simulink model "ex5"  (R2016b)
settings: Solver=ode23s  StartTime=0.0  StopTime=0.2  RelTol=1e-3
InitFcn:
  | ex5LIN_param
values from neighbouring files (symbols this model uses):
  A = [0 1; 0 -(dm/Jeq + Km*Kemf/(R*Jeq))]    [Lab3.m]    (also in Lab3_1.m; Lab3_2.m; Lab3_2_discrete_disg.m; Lab3_3.m)
  A1 = A3    (= 0.00180641577581)    [ex5LIN_param.m]    (also in param.m)
  A2 = A3    (= 0.00180641577581)    [ex5LIN_param.m]    (also in param.m)
  B = [0; Km/(R*Jeq)]    [Lab3.m]    (also in Lab3_1.m; Lab3_2.m; Lab3_2_discrete_disg.m; Lab3_3.m)
  beta = 2e9    (= 2000000000)    [ex5LIN_param.m]    (also in param.m)
  C = [1/n 0; 0 1/n]    [Lab3.m]    (also in Lab3_1.m; Lab3_2.m; Lab3_2_discrete_disg.m; Lab3_3.m)
  Cf1 = Cf    (= 6.32245521535e-13)    [ex5LIN_param.m]    (also in param.m)
  Cf2 = Cf    (= 6.32245521535e-13)    [ex5LIN_param.m]    (also in param.m)
  d = 0.001    [ex5LIN_param.m]    (also in param.m)
  D0 = zeros(3,2)    [ex5LIN.m]
  D_FBv = D_temp{1,1}    [ex5PID.m]
  D_FFv = D_temp{1,1}    [ex5PID.m]
  df = 200    [ex5LIN_param.m]    (also in param.m)
  fe0 = feINI(z)    [ex5LIN.m]
  m = 100    [ex5LIN_param.m]    (also in param.m)
  N_FBv = N_temp{1,1}    [ex5PID.m]
  N_FFv = N_temp{1,1}    [ex5PID.m]
  p1q0 = p1qINI(z)    [ex5LIN.m]
  p2q0 = p2qINI(z)    [ex5LIN.m]
  Ps = 20e6    (= 20000000)    [ex5LIN_param.m]    (also in param.m)
  Pt = 0    [ex5LIN_param.m]    (also in param.m)
  Rv = 1e-4    (= 0.0001)    [ex5LIN_param.m]    (also in param.m)
  smax = 0.7    [ex5LIN_param.m]    (also in param.m)
  vn = -0.01    [ex5LIN_param.m]    (also in param.m)
  vp = 0.01    [ex5LIN_param.m]    (also in param.m)
  vq0 = vqINI(z)    [ex5LIN.m]
  xvq0 = xvqINI(z)    [ex5LIN.m]
undefined symbols (not defined in the file or in its folder): D_C, D_FF, I_C, I_FF, K_C, K_FF, P_C, P_FF
libraries: simulink x4
settings Model: Creator=Philipp  LastModifiedBy=Philipp

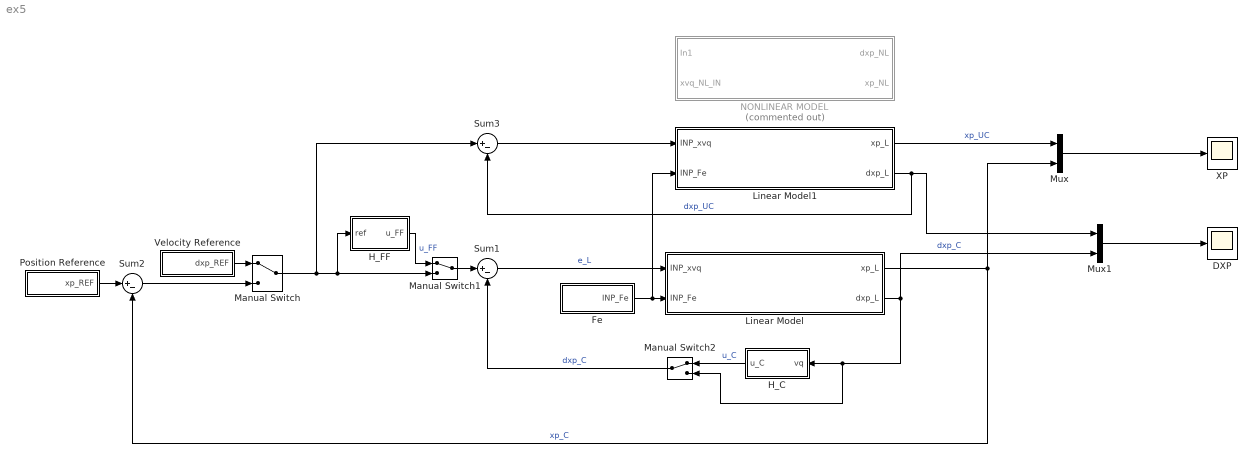
== system ex5 ==
  DXP : Scope
  Fe : Subsystem
  H_C : Subsystem
  H_FF : Subsystem
  Linear Model : Subsystem
  Linear Model1 : Subsystem
  Manual Switch : ManualSwitch
  Manual Switch1 : ManualSwitch
  Manual Switch2 : ManualSwitch
  Mux : Mux  Inputs=2
  Mux1 : Mux  Inputs=2
  NONLINEAR MODEL : Subsystem  Commented=on
  Position Reference : Subsystem
  Sum1 : Sum  Inputs=|+-
  Sum2 : Sum  Inputs=|+-
  Sum3 : Sum  Inputs=|+-
  Velocity Reference : Subsystem
  XP : Scope
  wires:
  H_FF/1(u_FF) -> Manual Switch1/1  "u_FF"
  H_C/1(u_C) -> Manual Switch2/1  "u_C"
  Sum2/1 -> Manual Switch/2
  Manual Switch/1 -> Sum3/1, H_FF/1(ref), Manual Switch1/2
  Manual Switch2/1 -> Sum1/2  "dxp_C"
  Manual Switch1/1 -> Sum1/1
  Position Reference/1(xp_REF) -> Sum2/1
  Velocity Reference/1(dxp_REF) -> Manual Switch/1
  Fe/1(INP_Fe) -> Linear Model1/2(INP_Fe), Linear Model/2(INP_Fe)
  Linear Model/2(dxp_L) -> Manual Switch2/2, H_C/1(vq), Mux1/2  "dxp_C"
  Linear Model/1(xp_L) -> Mux/2, Sum2/2  "xp_C"
  Sum1/1 -> Linear Model/1(INP_xvq)  "e_L"
  Linear Model1/1(xp_L) -> Mux/1  "xp_UC"
  Linear Model1/2(dxp_L) -> Sum3/2, Mux1/1  "dxp_UC"
  Mux1/1 -> DXP/1
  Mux/1 -> XP/1
  Sum3/1 -> Linear Model1/1(INP_xvq)

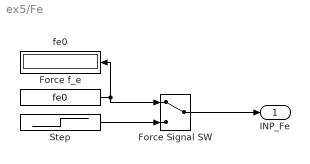
== system ex5/Fe ==
  Force Signal SW : ManualSwitch
  Force f_e : Constant  Value=fe0
  Step : Step  Time=0.12  After=0  SampleTime=0
  fe0 : Display
  INP_Fe : Outport
  wires:
  Force Signal SW/1 -> INP_Fe/1
  Force f_e/1 -> fe0/1, Force Signal SW/1
  Step/1 -> Force Signal SW/2

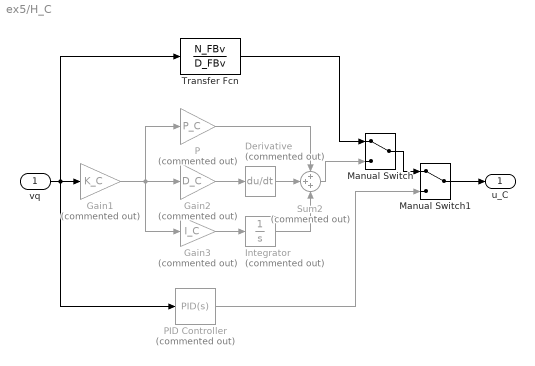
== system ex5/H_C ==
  vq : Inport
  Derivative : Derivative  Commented=on  CoefficientInTFapproximation=T_LPC
  Gain1 : Gain  Commented=on  Gain=K_C
  Gain2 : Gain  Commented=on  Gain=D_C
  Gain3 : Gain  Commented=on  Gain=I_C
  Integrator : Integrator  Commented=on
  Manual Switch : ManualSwitch
  Manual Switch1 : ManualSwitch
  P : Gain  Commented=on  Gain=P_C
  PID Controller : simulink/Continuous/PID Controller  Commented=on  Controller=PID  TimeDomain=Continuous-time  SampleTime=-1  IntegratorMethod=Forward Euler  FilterMethod=Forward Euler  Form=Parallel  UseFilter=on  ControllerParametersSource=internal  P=1  I=1  D=0  N=100  InitialConditionSource=internal  InitialConditionForIntegrator=0  InitialConditionForFilter=0  ExternalReset=none  LimitOutput=off  UpperSaturationLimit=inf  LowerSaturationLimit=-inf  LinearizeAsGain=on  AntiWindupMode=none  Kb=1  TrackingMode=off  Kt=1  PParamMin=[]  PParamMax=[]  IParamMin=[]  IParamMax=[]  DParamMin=[]  DParamMax=[]  NParamMin=[]  NParamMax=[]  KbParamMin=[]  KbParamMax=[]  KtParamMin=[]  KtParamMax=[]  POutMin=[]  POutMax=[]  IOutMin=[]  IOutMax=[]  DOutMin=[]  DOutMax=[]  NOutMin=[]  NOutMax=[]  KbOutMin=[]  KbOutMax=[]  KtOutMin=[]  KtOutMax=[]  IntegratorOutMin=[]  IntegratorOutMax=[]  FilterOutMin=[]  FilterOutMax=[]  SumOutMin=[]  SumOutMax=[]  SumI1OutMin=[]  SumI1OutMax=[]  SumI2OutMin=[]  SumI2OutMax=[]  SumI3OutMin=[]  SumI3OutMax=[]  SumDOutMin=[]  SumDOutMax=[]  SaturationOutMin=[]  SaturationOutMax=[]  IntegratorContinuousStateAttributes=''  IntegratorStateMustResolveToSignalObject=off  IntegratorRTWStateStorageClass=Auto  FilterContinuousStateAttributes=''  FilterStateMustResolveToSignalObject=off  FilterRTWStateStorageClass=Auto  DifferentiatorICPrevScaledInput=0  DifferentiatorOutMin=[]  DifferentiatorOutMax=[]
  Sum2 : Sum  Commented=on  Inputs=+++
  Transfer Fcn : TransferFcn  Numerator=N_FBv  Denominator=D_FBv
  u_C : Outport
  wires:
  Gain3/1 -> Integrator/1
  vq/1 -> PID Controller/1, Transfer Fcn/1, Gain1/1
  P/1 -> Sum2/1
  Derivative/1 -> Sum2/2
  Gain2/1 -> Derivative/1
  Integrator/1 -> Sum2/3
  Gain1/1 -> Gain3/1, Gain2/1, P/1
  Manual Switch1/1 -> u_C/1
  Manual Switch/1 -> Manual Switch1/1
  Transfer Fcn/1 -> Manual Switch/1
  Sum2/1 -> Manual Switch/2
  PID Controller/1 -> Manual Switch1/2

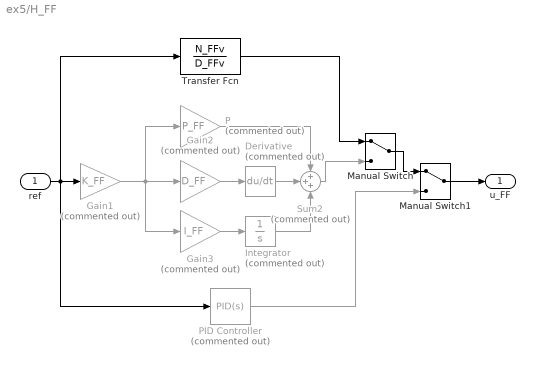
== system ex5/H_FF ==
  ref : Inport
  Derivative : Derivative  Commented=on  CoefficientInTFapproximation=T_LPFF
  Gain1 : Gain  Commented=on  Gain=K_FF
  Gain2 : Gain  Commented=on  Gain=D_FF
  Gain3 : Gain  Commented=on  Gain=I_FF
  Integrator : Integrator  Commented=on
  Manual Switch : ManualSwitch
  Manual Switch1 : ManualSwitch
  P : Gain  Commented=on  Gain=P_FF
  PID Controller : simulink/Continuous/PID Controller  Commented=on  Controller=PID  TimeDomain=Continuous-time  SampleTime=-1  IntegratorMethod=Forward Euler  FilterMethod=Forward Euler  Form=Parallel  UseFilter=on  ControllerParametersSource=internal  P=1  I=1  D=0  N=100  InitialConditionSource=internal  InitialConditionForIntegrator=0  InitialConditionForFilter=0  ExternalReset=none  LimitOutput=off  UpperSaturationLimit=inf  LowerSaturationLimit=-inf  LinearizeAsGain=on  AntiWindupMode=none  Kb=1  TrackingMode=off  Kt=1  PParamMin=[]  PParamMax=[]  IParamMin=[]  IParamMax=[]  DParamMin=[]  DParamMax=[]  NParamMin=[]  NParamMax=[]  KbParamMin=[]  KbParamMax=[]  KtParamMin=[]  KtParamMax=[]  POutMin=[]  POutMax=[]  IOutMin=[]  IOutMax=[]  DOutMin=[]  DOutMax=[]  NOutMin=[]  NOutMax=[]  KbOutMin=[]  KbOutMax=[]  KtOutMin=[]  KtOutMax=[]  IntegratorOutMin=[]  IntegratorOutMax=[]  FilterOutMin=[]  FilterOutMax=[]  SumOutMin=[]  SumOutMax=[]  SumI1OutMin=[]  SumI1OutMax=[]  SumI2OutMin=[]  SumI2OutMax=[]  SumI3OutMin=[]  SumI3OutMax=[]  SumDOutMin=[]  SumDOutMax=[]  SaturationOutMin=[]  SaturationOutMax=[]  IntegratorContinuousStateAttributes=''  IntegratorStateMustResolveToSignalObject=off  IntegratorRTWStateStorageClass=Auto  FilterContinuousStateAttributes=''  FilterStateMustResolveToSignalObject=off  FilterRTWStateStorageClass=Auto  DifferentiatorICPrevScaledInput=0  DifferentiatorOutMin=[]  DifferentiatorOutMax=[]
  Sum2 : Sum  Commented=on  Inputs=+++
  Transfer Fcn : TransferFcn  Numerator=N_FFv  Denominator=D_FFv
  u_FF : Outport
  wires:
  Gain3/1 -> Integrator/1
  ref/1 -> PID Controller/1, Transfer Fcn/1, Gain1/1
  P/1 -> Sum2/1
  Derivative/1 -> Sum2/2
  Gain2/1 -> Derivative/1
  Integrator/1 -> Sum2/3
  Gain1/1 -> Gain3/1, Gain2/1, P/1
  Manual Switch1/1 -> u_FF/1
  Manual Switch/1 -> Manual Switch1/1
  Transfer Fcn/1 -> Manual Switch/1
  Sum2/1 -> Manual Switch/2
  PID Controller/1 -> Manual Switch1/2

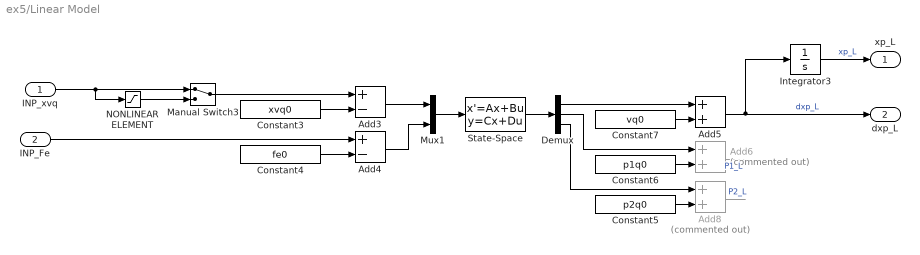
== system ex5/Linear Model ==
  INP_xvq : Inport
  INP_Fe : Inport  Port=2
  Add3 : Sum  Inputs=+-
  Add4 : Sum  Inputs=+-
  Add5 : Sum
  Add6 : Sum  Commented=on
  Add8 : Sum  Commented=on
  Constant3 : Constant  Value=xvq0
  Constant4 : Constant  Value=fe0
  Constant5 : Constant  Value=p2q0
  Constant6 : Constant  Value=p1q0
  Constant7 : Constant  Value=vq0
  Demux : Demux  Outputs=3
  Integrator3 : Integrator
  Manual Switch3 : ManualSwitch
  Mux1 : Mux  Inputs=2
  NONLINEAR ELEMENT : Saturate  UpperLimit=vp  LowerLimit=vn
  State-Space : StateSpace  A=A  B=B  C=C  D=D0  X0=0
  xp_L : Outport
  dxp_L : Outport  Port=2
  wires:
  Constant6/1 -> Add6/2
  Add4/1 -> Mux1/2
  Constant4/1 -> Add4/2
  Demux/2 -> Add6/1
  Demux/1 -> Add5/1
  Add5/1 -> Integrator3/1, dxp_L/1  "dxp_L"
  Mux1/1 -> State-Space/1
  Constant3/1 -> Add3/2
  Add3/1 -> Mux1/1
  Constant5/1 -> Add8/2
  Integrator3/1 -> xp_L/1  "xp_L"
  Constant7/1 -> Add5/2
  Demux/3 -> Add8/1
  INP_xvq/1 -> NONLINEAR ELEMENT/1, Manual Switch3/1
  State-Space/1 -> Demux/1
  INP_Fe/1 -> Add4/1
  Add6/1 -> ?  "P1_L"
  Add8/1 -> ?  "P2_L"
  Manual Switch3/1 -> Add3/1
  NONLINEAR ELEMENT/1 -> Manual Switch3/2

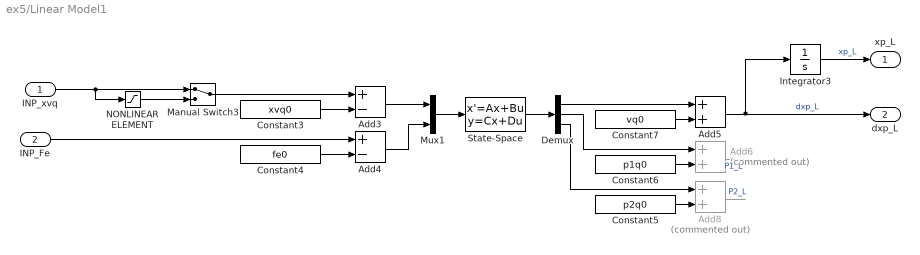
== system ex5/Linear Model1 ==
  INP_xvq : Inport
  INP_Fe : Inport  Port=2
  Add3 : Sum  Inputs=+-
  Add4 : Sum  Inputs=+-
  Add5 : Sum
  Add6 : Sum  Commented=on
  Add8 : Sum  Commented=on
  Constant3 : Constant  Value=xvq0
  Constant4 : Constant  Value=fe0
  Constant5 : Constant  Value=p2q0
  Constant6 : Constant  Value=p1q0
  Constant7 : Constant  Value=vq0
  Demux : Demux  Outputs=3
  Integrator3 : Integrator
  Manual Switch3 : ManualSwitch
  Mux1 : Mux  Inputs=2
  NONLINEAR ELEMENT : Saturate  UpperLimit=vp  LowerLimit=vn
  State-Space : StateSpace  A=A  B=B  C=C  D=D0  X0=0
  xp_L : Outport
  dxp_L : Outport  Port=2
  wires:
  Constant6/1 -> Add6/2
  Add4/1 -> Mux1/2
  Constant4/1 -> Add4/2
  Demux/2 -> Add6/1
  Demux/1 -> Add5/1
  Add5/1 -> Integrator3/1, dxp_L/1  "dxp_L"
  Mux1/1 -> State-Space/1
  Constant3/1 -> Add3/2
  Add3/1 -> Mux1/1
  Constant5/1 -> Add8/2
  Integrator3/1 -> xp_L/1  "xp_L"
  Constant7/1 -> Add5/2
  Demux/3 -> Add8/1
  INP_xvq/1 -> NONLINEAR ELEMENT/1, Manual Switch3/1
  State-Space/1 -> Demux/1
  INP_Fe/1 -> Add4/1
  Add6/1 -> ?  "P1_L"
  Add8/1 -> ?  "P2_L"
  Manual Switch3/1 -> Add3/1
  NONLINEAR ELEMENT/1 -> Manual Switch3/2

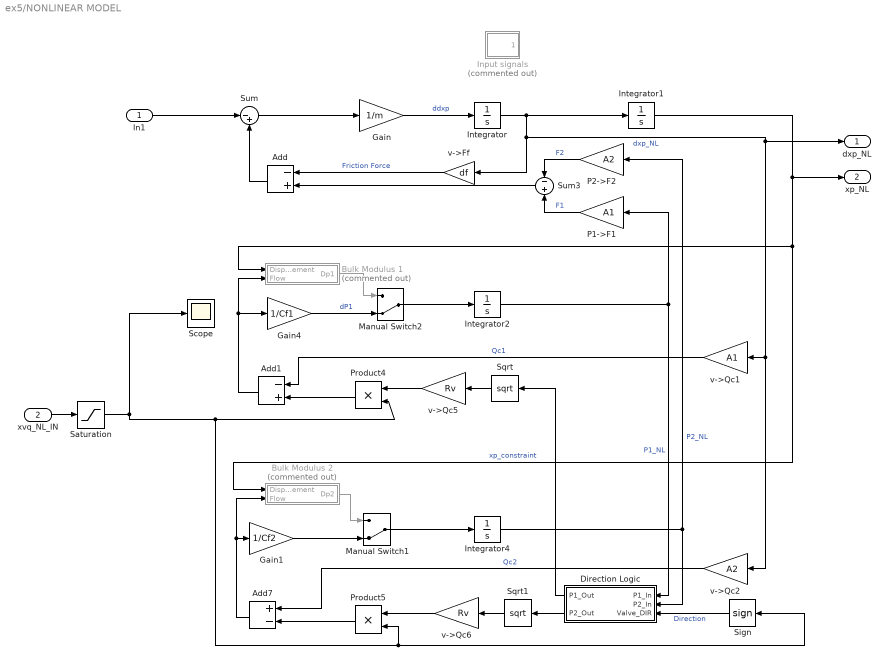
== system ex5/NONLINEAR MODEL ==
  In1 : Inport
  xvq_NL_IN : Inport  Port=2
  Add : Sum  Inputs=-+
  Add1 : Sum  Inputs=-+
  Add7 : Sum  Inputs=+-
  Bulk Modulus 1 : Subsystem  Commented=on
  Bulk Modulus 2 : Subsystem  Commented=on
  Direction Logic : Subsystem
  Gain : Gain  Gain=1/m
  Gain1 : Gain  Gain=1/Cf2
  Gain4 : Gain  Gain=1/Cf1
  Input signals : Subsystem  Commented=on
  Integrator : Integrator
  Integrator1 : Integrator  LimitOutput=on  UpperSaturationLimit=(smax/2-d)  LowerSaturationLimit=-(smax/2-d)
  Integrator2 : Integrator
  Integrator4 : Integrator
  Manual Switch1 : ManualSwitch  CurrentSetting=0
  Manual Switch2 : ManualSwitch  CurrentSetting=0
  P1->F1 : Gain  Gain=A1
  P2->F2 : Gain  Gain=A2
  Product4 : Product
  Product5 : Product
  Saturation : Saturate  UpperLimit=vp  LowerLimit=vn
  Scope : Scope
  Sign : Signum
  Sqrt : Sqrt  SaturateOnIntegerOverflow=on
  Sqrt1 : Sqrt  SaturateOnIntegerOverflow=on
  Sum : Sum  Inputs=|-+
  Sum3 : Sum  Inputs=-+
  v->Ff : Gain  Gain=df
  v->Qc1 : Gain  Gain=A1
  v->Qc2 : Gain  Gain=A2
  v->Qc5 : Gain  Gain=Rv
  v->Qc6 : Gain  Gain=Rv
  dxp_NL : Outport
  xp_NL : Outport  Port=2
  wires:
  Sign/1 -> Direction Logic/3(Valve_DIR)  "Direction"
  v->Qc5/1 -> Product4/1
  Add/1 -> Sum/2
  Sum3/1 -> Add/2
  Bulk Modulus 1/1(Dp1) -> Manual Switch2/1
  Sum/1 -> Gain/1
  Add1/1 -> Bulk Modulus 1/2(Flow), Gain4/1
  P1->F1/1 -> Sum3/2  "F1"
  P2->F2/1 -> Sum3/1  "F2"
  Add7/1 -> Bulk Modulus 2/2(Flow), Gain1/1
  Integrator2/1 -> Direction Logic/1(P1_In), P1->F1/1  "P1_NL"
  Integrator4/1 -> P2->F2/1, Direction Logic/2(P2_In)  "P2_NL"
  Manual Switch1/1 -> Integrator4/1
  Sqrt/1 -> v->Qc5/1
  Integrator1/1 -> xp_NL/1, Bulk Modulus 2/1(Displacement), Bulk Modulus 1/1(Displacement)  "xp_constraint"
  Bulk Modulus 2/1(Dp2) -> Manual Switch1/1
  Direction Logic/1(P1_Out) -> Sqrt/1
  v->Qc2/1 -> Add7/1  "Qc2"
  Sqrt1/1 -> v->Qc6/1
  v->Ff/1 -> Add/1  "Friction Force"
  Direction Logic/2(P2_Out) -> Sqrt1/1
  Product4/1 -> Add1/2
  Gain4/1 -> Manual Switch2/2  "dP1"
  Manual Switch2/1 -> Integrator2/1
  Product5/1 -> Add7/2
  v->Qc6/1 -> Product5/1
  Gain/1 -> Integrator/1  "ddxp"
  Gain1/1 -> Manual Switch1/2
  Integrator/1 -> Integrator1/1, dxp_NL/1, v->Qc2/1, v->Qc1/1, v->Ff/1  "dxp_NL"
  v->Qc1/1 -> Add1/1  "Qc1"
  Saturation/1 -> Product4/2, Product5/2, Sign/1, Scope/1
  xvq_NL_IN/1 -> Saturation/1
  In1/1 -> Sum/1

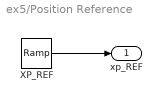
== system ex5/Position Reference ==
  XP_REF : simulink/Sources/Ramp  slope=1  start=0  X0=0
  xp_REF : Outport
  wires:
  XP_REF/1 -> xp_REF/1

== system ex5/Velocity Reference ==
  DXP_REF : DiscretePulseGenerator  PulseType=Time based  Amplitude=0.5  Period=1  PulseWidth=50
  dxp_REF : Outport
  wires:
  DXP_REF/1 -> dxp_REF/1  "dxp_Ref"

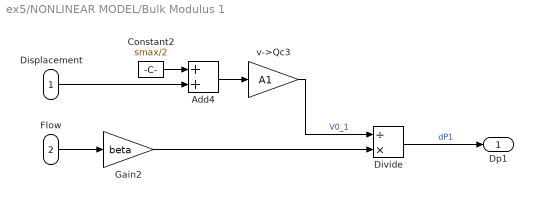
== system ex5/NONLINEAR MODEL/Bulk Modulus 1 ==
  Displacement : Inport
  Flow : Inport  Port=2
  Add4 : Sum
  Constant2 : Constant  Value=smax/2
  Divide : Product  Inputs=/*
  Gain2 : Gain  Gain=beta
  v->Qc3 : Gain  Gain=A1
  Dp1 : Outport
  wires:
  Flow/1 -> Gain2/1
  Displacement/1 -> Add4/2
  Constant2/1 -> Add4/1
  Divide/1 -> Dp1/1  "dP1"
  v->Qc3/1 -> Divide/1  "V0_1"
  Gain2/1 -> Divide/2
  Add4/1 -> v->Qc3/1

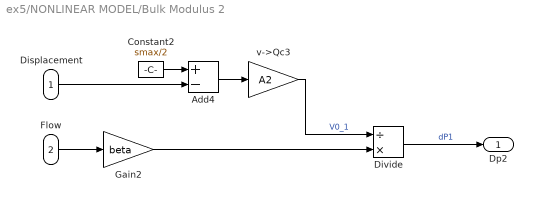
== system ex5/NONLINEAR MODEL/Bulk Modulus 2 ==
  Displacement : Inport
  Flow : Inport  Port=2
  Add4 : Sum  Inputs=+-
  Constant2 : Constant  Value=smax/2
  Divide : Product  Inputs=/*
  Gain2 : Gain  Gain=beta
  v->Qc3 : Gain  Gain=A2
  Dp2 : Outport
  wires:
  Flow/1 -> Gain2/1
  Displacement/1 -> Add4/2
  Constant2/1 -> Add4/1
  Divide/1 -> Dp2/1  "dP1"
  v->Qc3/1 -> Divide/1  "V0_1"
  Gain2/1 -> Divide/2
  Add4/1 -> v->Qc3/1

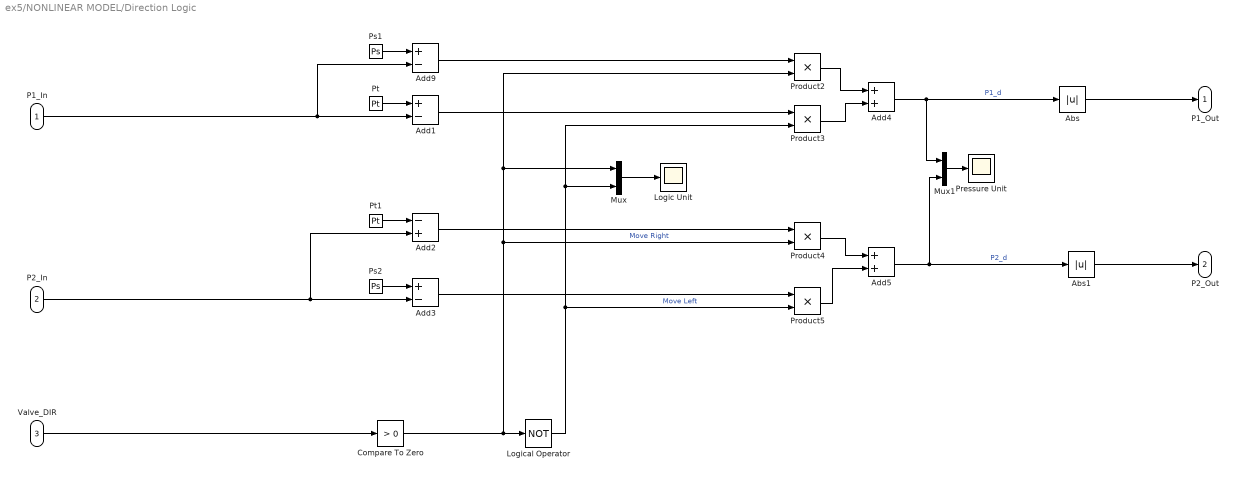
== system ex5/NONLINEAR MODEL/Direction Logic ==
  P1_In : Inport
  P2_In : Inport  Port=2
  Valve_DIR : Inport  Port=3
  Abs : Abs  ZeroCross=off
  Abs1 : Abs
  Add1 : Sum  Inputs=+-
  Add2 : Sum  Inputs=-+
  Add3 : Sum  Inputs=+-
  Add4 : Sum
  Add5 : Sum
  Add9 : Sum  Inputs=+-
  Compare To Zero : simulink/Logic and Bit Operations/Compare To Zero  relop=>  OutDataTypeStr=boolean
  Logic Unit : Scope
  Logical Operator : Logic  Operator=NOT  AllPortsSameDT=off  OutDataTypeStr=boolean
  Mux : Mux  Inputs=2
  Mux1 : Mux  Inputs=2
  Pressure Unit : Scope
  Product{2..5} (4 alike) : Product
  Ps1 : Constant  Value=Ps
  Ps2 : Constant  Value=Ps
  Pt : Constant  Value=Pt
  Pt1 : Constant  Value=Pt
  P1_Out : Outport
  P2_Out : Outport  Port=2
  wires:
  Valve_DIR/1 -> Compare To Zero/1
  Compare To Zero/1 -> Mux/1, Product2/2, Product4/2, Logical Operator/1  "Move Right"
  Logical Operator/1 -> Mux/2, Product3/2, Product5/2  "Move Left"
  Add9/1 -> Product2/1
  Ps1/1 -> Add9/1
  P1_In/1 -> Add1/2, Add9/2
  Add1/1 -> Product3/1
  Add3/1 -> Product5/1
  Ps2/1 -> Add3/1
  P2_In/1 -> Add2/2, Add3/2
  Add2/1 -> Product4/1
  Pt1/1 -> Add2/1
  Pt/1 -> Add1/1
  Product2/1 -> Add4/1
  Product3/1 -> Add4/2
  Product4/1 -> Add5/1
  Product5/1 -> Add5/2
  Add4/1 -> Abs/1, Mux1/1  "P1_d"
  Abs/1 -> P1_Out/1
  Abs1/1 -> P2_Out/1
  Add5/1 -> Abs1/1, Mux1/2  "P2_d"
  Mux/1 -> Logic Unit/1
  Mux1/1 -> Pressure Unit/1

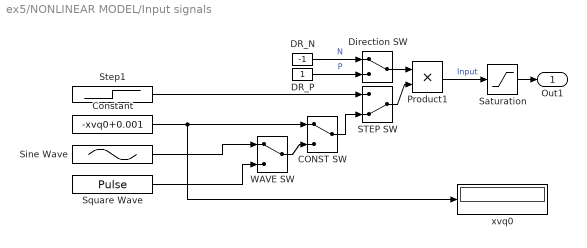
== system ex5/NONLINEAR MODEL/Input signals ==
  CONST SW : ManualSwitch
  Constant : Constant  Value=-xvq0+0.001
  DR_N : Constant  Value=-1
  "DR_P " : Constant
  Direction SW : ManualSwitch
  Product1 : Product
  STEP SW : ManualSwitch  CurrentSetting=0
  Saturation : Saturate  UpperLimit=vp  LowerLimit=vn
  Sine Wave : Sin  Amplitude=xvq0  Frequency=2*pi*1/2  Phase=pi/2  SampleTime=0
  Square Wave : DiscretePulseGenerator  PulseType=Time based  Amplitude=0.0001  PulseWidth=50
  Step1 : Step  Time=0  After=0.005  SampleTime=0
  WAVE SW : ManualSwitch
  xvq0 : Display
  Out1 : Outport
  wires:
  Saturation/1 -> Out1/1
  WAVE SW/1 -> CONST SW/2
  DR_N/1 -> Direction SW/1  "N"
  Step1/1 -> STEP SW/1
  Product1/1 -> Saturation/1  "Input"
  CONST SW/1 -> STEP SW/2
  Direction SW/1 -> Product1/1
  STEP SW/1 -> Product1/2
  Sine Wave/1 -> WAVE SW/1
  "DR_P "/1 -> Direction SW/2  "P"
  Square Wave/1 -> WAVE SW/2
  Constant/1 -> xvq0/1, CONST SW/1
